simulink model "skidPadSimulation_MPC_Basic"  (R2026a)
settings: Solver=VariableStepAuto  StopTime=80
InitFcn:
  | skidpad_init
values from neighbouring files (symbols this model uses):
  waypoints = [path_data.x_norm, path_data.y_norm, path_data.psi]    [skidpad_init.m]
undefined symbols (not defined in the file or in its folder): ic
settings Model: Creator=lholliday  LastModifiedBy=lholliday

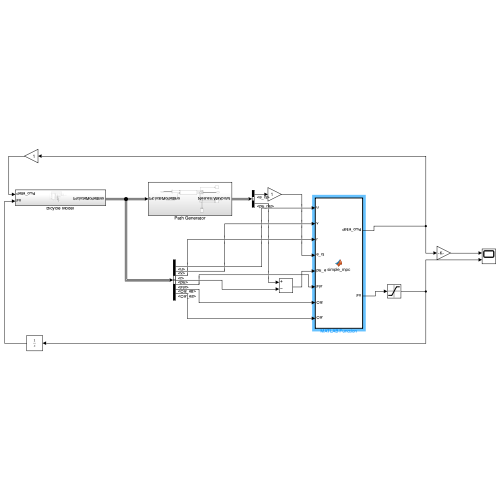
[thumbnail: Simulink's stored preview of the top-level diagram]
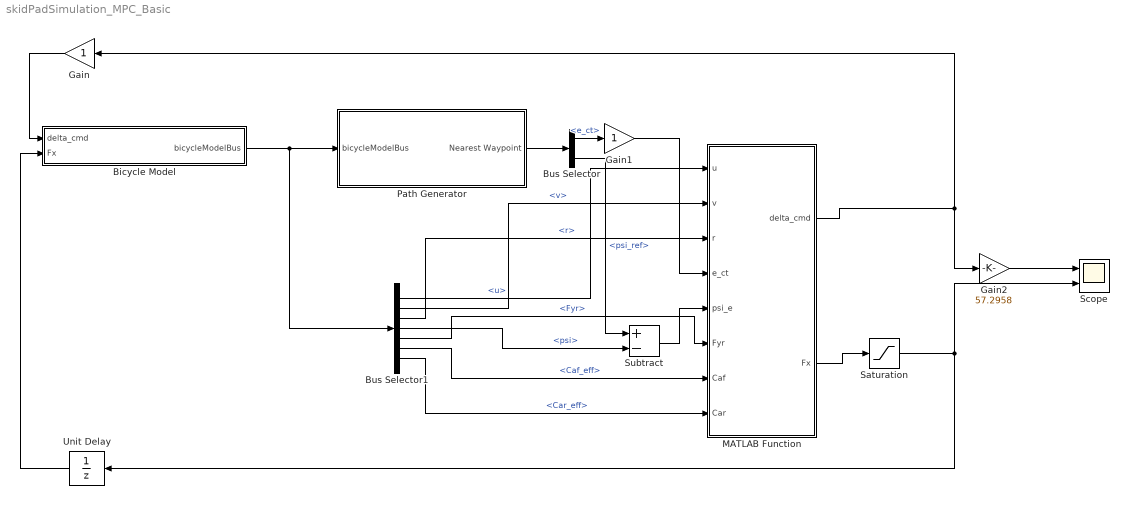
== system skidPadSimulation_MPC_Basic ==
  Bicycle Model : Subsystem
  Bus Selector : BusSelector  OutputSignals=e_ct,psi_ref
  Bus Selector1 : BusSelector  OutputSignals=u,v,r,psi,Fyr,Caf_eff,Car_eff
  Gain : Gain
  Gain1 : Gain
  Gain2 : Gain  Gain=57.2958
  MATLAB Function : MATLAB Function  TreatAsAtomicUnit=on
  Path Generator : Subsystem
  Saturation : Saturate  UpperLimit=2000  LowerLimit=-2000
  Scope : Scope  NumInputPorts=2
      settings: ActiveDisplayYMinimum=-62.500022347760442  ActiveDisplayYMaximum=62.500022347760442  DataLoggingVariableName=ScopeData8
  Subtract : Sum  Inputs=+-
  Unit Delay : UnitDelay  SampleTime=0.01
  wires:
  Path Generator/1(Nearest Waypoint) -> Bus Selector/1
  Bicycle Model/1(bicycleModelBus) -> Path Generator/1(bicycleModelBus), Bus Selector1/1
  Bus Selector/1 -> Gain1/1  "<e_ct>"
  Bus Selector/2 -> Subtract/1  "<psi_ref>"
  Bus Selector1/4 -> Subtract/2  "<psi>"
  Subtract/1 -> MATLAB Function/5(psi_e)
  Bus Selector1/1 -> MATLAB Function/1(u)  "<u>"
  Bus Selector1/2 -> MATLAB Function/2(v)  "<v>"
  Bus Selector1/3 -> MATLAB Function/3(r)  "<r>"
  MATLAB Function/2(Fx) -> Saturation/1
  Bus Selector1/5 -> MATLAB Function/6(Fyr)  "<Fyr>"
  Saturation/1 -> Scope/2, Unit Delay/1
  Gain/1 -> Bicycle Model/1(delta_cmd)
  Gain1/1 -> MATLAB Function/4(e_ct)
  MATLAB Function/1(delta_cmd) -> Gain/1, Gain2/1
  Gain2/1 -> Scope/1
  Unit Delay/1 -> Bicycle Model/2(Fx)
  Bus Selector1/6 -> MATLAB Function/7(Caf)  "<Caf_eff>"
  Bus Selector1/7 -> MATLAB Function/8(Car)  "<Car_eff>"

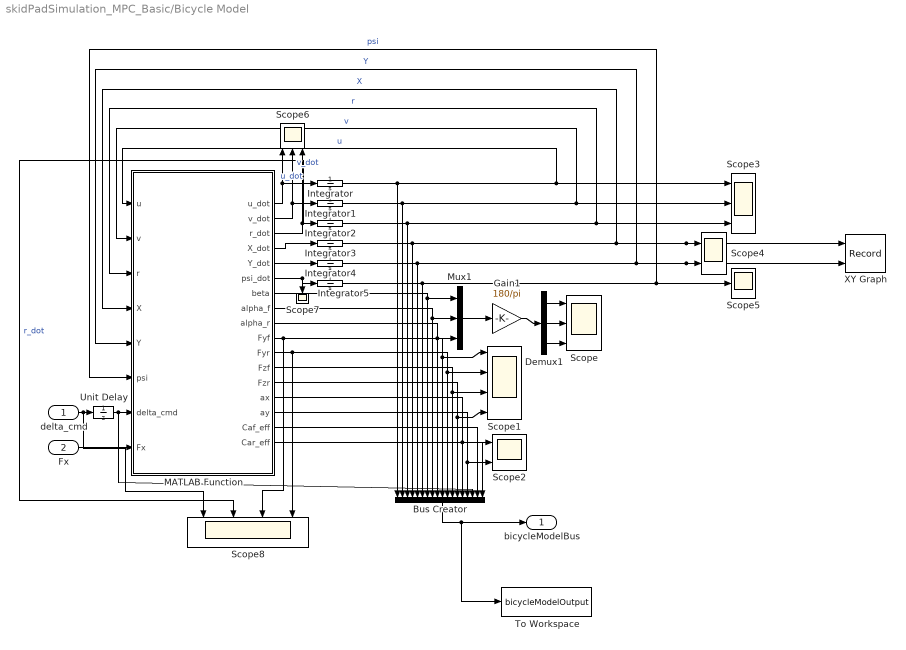
== system skidPadSimulation_MPC_Basic/Bicycle Model ==
  delta_cmd : Inport
  Fx : Inport  Port=2
  Bus Creator : BusCreator  Inputs=18
  Demux1 : Demux  Outputs=3
  Gain1 : Gain  Gain=180/pi
  Integrator : Integrator  InitialCondition=1
  Integrator1 : Integrator
  Integrator2 : Integrator
  Integrator3 : Integrator  InitialCondition=ic.X
  Integrator4 : Integrator  InitialCondition=ic.Y
  Integrator5 : Integrator
  MATLAB Function : MATLAB Function  TreatAsAtomicUnit=on
  Mux1 : Mux  Inputs=3
  Scope : Scope  NumInputPorts=3
      settings: ActiveDisplayYMinimum=-4.6519125249933184  ActiveDisplayYMaximum=6.7259914561440342
  Scope1 : Scope  NumInputPorts=4
      settings: ActiveDisplayYMinimum=-8171.7683750096539  ActiveDisplayYMaximum=8472.1779002535986
  Scope2 : Scope  NumInputPorts=2
      settings: ActiveDisplayYMinimum=-9.4735919080060764  ActiveDisplayYMaximum=10.384655851195211  DataLoggingVariableName=ScopeData2
  Scope3 : Scope  NumInputPorts=3
      settings: ActiveDisplayYMinimum=-0.57485772650992173  ActiveDisplayYMaximum=15.1737195385893  DataLoggingVariableName=ScopeData3
  Scope4 : Scope  NumInputPorts=2
      settings: ActiveDisplayYMinimum=-1031.663648785918  ActiveDisplayYMaximum=2103.4580897021219  DataLoggingVariableName=ScopeData4
  Scope5 : Scope
      settings: ActiveDisplayYMinimum=-1  ActiveDisplayYMaximum=1  DataLoggingVariableName=ScopeData5
  Scope6 : Scope  NumInputPorts=3
      settings: ActiveDisplayYMinimum=-0.28609045005768552  ActiveDisplayYMaximum=2.7161396379868852  DataLoggingVariableName=ScopeData6
  Scope7 : Scope
      settings: ActiveDisplayYMinimum=-1.109696536806452  ActiveDisplayYMaximum=1.2916224827655673  DataLoggingVariableName=ScopeData10
  Scope8 : Scope  NumInputPorts=4
      settings: ActiveDisplayYMinimum=-0.43633231299858238  ActiveDisplayYMaximum=0.43633231299858238  DataLoggingVariableName=ScopeData11
  To Workspace : ToWorkspace  VariableName=bicycleModelOutput  SaveFormat=Timeseries  SampleTime=-1
  Unit Delay : UnitDelay  SampleTime=0.01
  XY Graph : Record  NumPorts=2.0  FileSettingsInternal="{\"entries\":[{\"content\":{\"excelSettings\":{\"content\":{},\"type\":\"Streamout.ExcelSettings\"},\"parquetSettings\":{\"content\":{},\"type\":\"Streamout.ParquetSettings\"}},\"type\":\"Streamout.FileSettingStorage\",\"uuid\":\"\"}],\"packageUris\":[\"http:\\/\\/schema.mathworks.com\\/mf0\\/streamout_blocks\\/R2020a\"],\"version\":\"1.0\"}"  FrameSettings=[0, 0]  Layout=[1 1]  SignalsInternal="{\"entries\":[{\"content\":{\"signals\":[{\"content\":{\"blockPath\":[],\"dimensions\":[1],\"domain\":\"\",\"lineColor\":\"#a2142f\",\"plots\":[ 1 ],\"port\":1,\"sid\":[\"\"],\"signalID\":1,\"signalName\":\"X\"},\"type\":\"RecordBlkView.Signal\",\"uuid\":\"\"},{\"content\":{\"blockPath\":[],\"dimensions\":[1],\"domain\":\"\",\"lineColor\":\"#139fff\",\"plots\":[ 1 ],\"port\":2,\"sid\":[\"\"],\"signalID\":2,\"signalName\":\"Y\"},\"type\":\"RecordBlkView.Signal\",\"uuid\":\"\"}]},\"type\":\"RecordBlkView.InputSignals\",\"uuid\":\"\"}],\"packageUris\":[\"http:\\/\\/schema.mathworks.com\\/mf0\\/streamout_blocks\\/R2020a\"],\"version\":\"1.0\"}"  VisualizationBindings="{\"xyplotplugin\":{\"info\":[{\"series\":[{\"bindingParametersList\":[{\"parameter\":\"X-Axis\",\"signalID\":1,\"signalName\":\"X\"},{\"parameter\":\"Y-Axis\",\"signalID\":2,\"signalName\":\"Y\"}],\"seriesID\":0}],\"subplotID\":1}]}}"  CompatibilityTag=XY
  bicycleModelBus : Outport
  wires:
  ? -> ?
  MATLAB Function/2(v_dot) -> Scope6/2, Integrator1/1  "v_dot"
  MATLAB Function/3(r_dot) -> Scope8/2, Scope6/3, Integrator2/1  "r_dot"
  MATLAB Function/4(X_dot) -> Integrator3/1
  MATLAB Function/5(Y_dot) -> Integrator4/1
  MATLAB Function/6(psi_dot) -> Integrator5/1, Scope7/1
  MATLAB Function/1(u_dot) -> Scope6/1, Integrator/1  "u_dot"
  Integrator1/1 -> Scope3/2, MATLAB Function/2(v), Bus Creator/2  "v"
  Integrator2/1 -> Scope3/3, MATLAB Function/3(r), Bus Creator/3  "r"
  Integrator3/1 -> MATLAB Function/4(X), XY Graph/1, Scope4/1, Bus Creator/4  "X"
  Integrator4/1 -> MATLAB Function/5(Y), XY Graph/2, Scope4/2, Bus Creator/5  "Y"
  Integrator5/1 -> MATLAB Function/6(psi), Scope5/1, Bus Creator/6  "psi"
  MATLAB Function/8(alpha_f) -> Bus Creator/8, Mux1/2
  MATLAB Function/7(beta) -> Bus Creator/7, Mux1/1
  MATLAB Function/10(Fyf) -> Scope8/3, Bus Creator/10, Scope1/1
  MATLAB Function/12(Fzf) -> Bus Creator/12, Scope1/3
  MATLAB Function/13(Fzr) -> Bus Creator/13, Scope1/4
  MATLAB Function/15(ay) -> Scope2/2, Bus Creator/15
  MATLAB Function/14(ax) -> Scope2/1, Bus Creator/14
  Fx/1 -> MATLAB Function/8(Fx)
  Bus Creator/1 -> To Workspace/1, bicycleModelBus/1
  Integrator/1 -> Scope3/1, MATLAB Function/1(u), Bus Creator/1  "u"
  delta_cmd/1 -> Scope8/1, Unit Delay/1
  Unit Delay/1 -> Bus Creator/16, MATLAB Function/7(delta_cmd)
  Gain1/1 -> Demux1/1
  Mux1/1 -> Gain1/1
  Demux1/1 -> Scope/1
  Demux1/2 -> Scope/2
  Demux1/3 -> Scope/3
  MATLAB Function/11(Fyr) -> Scope8/4, Bus Creator/11, Scope1/2
  MATLAB Function/9(alpha_r) -> Bus Creator/9, Mux1/3
  MATLAB Function/16(Caf_eff) -> Bus Creator/17
  MATLAB Function/17(Car_eff) -> Bus Creator/18

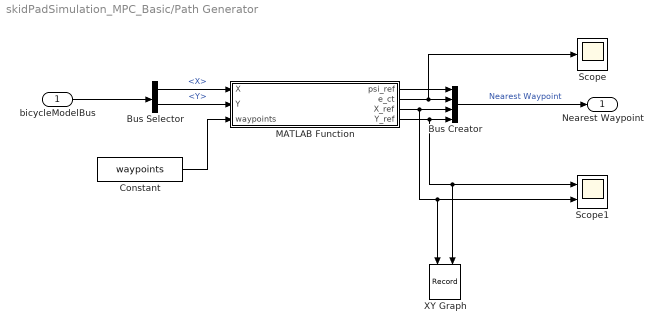
== system skidPadSimulation_MPC_Basic/Path Generator ==
  bicycleModelBus : Inport
  Bus Creator : BusCreator  Inputs=4
  Bus Selector : BusSelector  OutputSignals=X,Y
  Constant : Constant  Value=waypoints
  MATLAB Function : MATLAB Function  TreatAsAtomicUnit=on
  Scope : Scope
      settings: ActiveDisplayYMinimum=-362.12936641992621  ActiveDisplayYMaximum=253.81612411681579  DataLoggingVariableName=ScopeData7
  Scope1 : Scope  NumInputPorts=2
      settings: ActiveDisplayYMinimum=-362.12936641992621  ActiveDisplayYMaximum=253.81612411681579  DataLoggingVariableName=ScopeData9
  XY Graph : Record  NumPorts=2.0  FileSettingsInternal="{\"entries\":[{\"content\":{\"excelSettings\":{\"content\":{},\"type\":\"Streamout.ExcelSettings\"},\"parquetSettings\":{\"content\":{},\"type\":\"Streamout.ParquetSettings\"}},\"type\":\"Streamout.FileSettingStorage\",\"uuid\":\"\"}],\"packageUris\":[\"http:\\/\\/schema.mathworks.com\\/mf0\\/streamout_blocks\\/R2020a\"],\"version\":\"1.0\"}"  FrameSettings=[0, 0]  Layout=[1 1]  SignalsInternal="{\"entries\":[{\"content\":{\"signals\":[{\"content\":{\"blockPath\":[],\"dimensions\":[1],\"domain\":\"\",\"lineColor\":\"#a2142f\",\"plots\":[ 1 ],\"port\":1,\"sid\":[\"\"],\"signalID\":1,\"signalName\":\"MATLAB Function:3\"},\"type\":\"RecordBlkView.Signal\",\"uuid\":\"\"},{\"content\":{\"blockPath\":[],\"dimensions\":[1],\"domain\":\"\",\"lineColor\":\"#139fff\",\"plots\":[ 1 ],\"port\":2,\"sid\":[\"\"],\"signalID\":2,\"signalName\":\"MATLAB Function:4\"},\"type\":\"RecordBlkView.Signal\",\"uuid\":\"\"}]},\"type\":\"RecordBlkView.InputSignals\",\"uuid\":\"\"}],\"packageUris\":[\"http:\\/\\/schema.mathworks.com\\/mf0\\/streamout_blocks\\/R2020a\"],\"version\":\"1.0\"}"  VisualizationBindings="{\"xyplotplugin\":{\"info\":[{\"series\":[{\"bindingParametersList\":[{\"parameter\":\"X-Axis\",\"signalID\":1,\"signalName\":\"MATLAB Function:3\"},{\"parameter\":\"Y-Axis\",\"signalID\":2,\"signalName\":\"MATLAB Function:4\"}],\"seriesID\":0}],\"subplotID\":1}]}}"  CompatibilityTag=XY
  Nearest Waypoint : Outport
  wires:
  bicycleModelBus/1 -> Bus Selector/1
  Bus Selector/1 -> MATLAB Function/1(X)  "<X>"
  Bus Selector/2 -> MATLAB Function/2(Y)  "<Y>"
  MATLAB Function/1(psi_ref) -> Bus Creator/1
  MATLAB Function/2(e_ct) -> Scope/1, Bus Creator/2
  MATLAB Function/3(X_ref) -> XY Graph/1, Scope1/2, Bus Creator/3
  MATLAB Function/4(Y_ref) -> XY Graph/2, Scope1/1, Bus Creator/4
  Bus Creator/1 -> Nearest Waypoint/1  "Nearest Waypoint"
  Constant/1 -> MATLAB Function/3(waypoints)

== matlab function skidPadSimulation_MPC_Basic/Path Generator/MATLAB Function ==
  settings: updateMethod=DISCRETE
  data: X input; psi_ref output; Y input; e_ct output; X_ref output; Y_ref output; waypoints input
function [psi_ref, e_ct, X_ref, Y_ref] = nearest_waypoint(X, Y, waypoints)

% NEAREST_WAYPOINT  Robust path-relative error calculation.
%
% Improvements over basic nearest-point search:
%   1. Persistent forward-only progress index - prevents the index
%      jumping backward or matching a point from a previous lap.
%   2. Bounded local search window around the last known progress -
%      cheaper than scanning all waypoints, and structurally prevents
%      far-away false matches.
%   3. True nearest-point-on-SEGMENT projection (not nearest waypoint) -
%      gives continuous, sub-waypoint-spacing accuracy for e_ct.
%   4. Linear interpolation of psi_ref between the two bracketing
%      waypoints, rather than a discrete jump at each waypoint.
%
% INPUTS:
%   X, Y      - current vehicle position [m]
%   waypoints - [N x 3] array of [X_wp, Y_wp, psi_wp]
%
% OUTPUTS:
%   psi_ref - interpolated path heading at the nearest point [rad]
%   e_ct    - signed cross track error, positive = left of path [m]
%   X_ref   - nearest point ON THE PATH (segment-projected, not a
%             discrete waypoint) [m]
%   Y_ref   - as above [m]

persistent prog_idx
if isempty(prog_idx)
    prog_idx = int32(1);
end

n = int32(size(waypoints, 1));

% -------------------------------------------------------------------
% Step 1: bounded forward search for the nearest waypoint, starting
% from last known progress. Allows a small backward window in case the
% car is briefly behind its last matched point (e.g. low speed,
% momentary correction), but never searches far enough back to match
% a previous lap.
% -------------------------------------------------------------------
back_window = int32(5);
fwd_window  = int32(40);

i_start = max(int32(1), prog_idx - back_window);
i_end   = min(n, prog_idx + fwd_window);

search_idx = i_start:i_end;
dx = waypoints(search_idx,1) - X;
dy = waypoints(search_idx,2) - Y;
dist_sq = dx.^2 + dy.^2;

[~, local_min] = min(dist_sq);
nearest_idx = search_idx(local_min);

prog_idx = nearest_idx;   % advance persistent progress

% -------------------------------------------------------------------
% Step 2: project the vehicle position onto the path SEGMENT either
% side of nearest_idx (whichever segment it actually falls within),
% rather than just using the nearest discrete waypoint. This removes
% most of the e_ct discretisation error from waypoint spacing.
% -------------------------------------------------------------------
idx_prev = max(int32(1), nearest_idx - int32(1));
idx_next = min(n,        nearest_idx + int32(1));

[Xp1, Yp1, dproj1, t1] = project_to_segment(X, Y, waypoints(idx_prev,1:2), waypoints(nearest_idx,1:2));
[Xp2, Yp2, dproj2, t2] = project_to_segment(X, Y, waypoints(nearest_idx,1:2), waypoints(idx_next,1:2));

if dproj1 <= dproj2
    X_ref = Xp1;
    Y_ref = Yp1;
    psi_a = waypoints(idx_prev, 3);
    psi_b = waypoints(nearest_idx, 3);
    t     = t1;
else
    X_ref = Xp2;
    Y_ref = Yp2;
    psi_a = waypoints(nearest_idx, 3);
    psi_b = waypoints(idx_next, 3);
    t     = t2;
end

% -------------------------------------------------------------------
% Step 3: interpolate heading between the two bracketing waypoints
% (shortest-angle interpolation to avoid wraparound issues near +-pi)
% -------------------------------------------------------------------
dpsi = atan2(sin(psi_b - psi_a), cos(psi_b - psi_a));
psi_ref = psi_a + t * dpsi;
psi_ref = atan2(sin(psi_ref), cos(psi_ref));   % wrap to [-pi, pi]

% -------------------------------------------------------------------
% Step 4: signed cross track error using the interpolated path heading
% -------------------------------------------------------------------
dx_ref = X - X_ref;
dy_ref = Y - Y_ref;
e_ct   = -sin(psi_ref)*dx_ref + cos(psi_ref)*dy_ref;

end


function [Xp, Yp, dist_sq, t] = project_to_segment(X, Y, P1, P2)
% Project point (X,Y) onto the segment P1->P2, clamped to [0,1].
% Returns the projected point, squared distance to it, and the
% fractional position t along the segment (used for interpolation).

vx = P2(1) - P1(1);
vy = P2(2) - P1(2);
seg_len_sq = vx^2 + vy^2;

if seg_len_sq < 1e-9
    % Degenerate segment (coincident points) - just use P1
    Xp = P1(1);
    Yp = P1(2);
    t  = 0;
else
    t = ((X - P1(1))*vx + (Y - P1(2))*vy) / seg_len_sq;
    t = max(0, min(1, t));
    Xp = P1(1) + t*vx;
    Yp = P1(2) + t*vy;
end

dist_sq = (X - Xp)^2 + (Y - Yp)^2;

end

== matlab function skidPadSimulation_MPC_Basic/Bicycle Model/MATLAB Function ==
  data: u_dot output; v_dot output; u input; v input; r_dot output; X_dot output; r input; X input; Y input; psi input; delta_cmd input; Fx input; Y_dot output; psi_dot output; beta output; alpha_f output; alpha_r output; Fyf output; Fyr output; Fzf output; Fzr output; ax output; ay output; Caf_eff output; Car_eff output
function [u_dot, v_dot, r_dot, X_dot, Y_dot, psi_dot, ...
          beta, alpha_f, alpha_r, Fyf, Fyr, Fzf, Fzr, ax, ay, Caf_eff, Car_eff] = ...
    bicycle_model_plant(u, v, r, X, Y, psi, delta_cmd, Fx)

% BICYCLE_MODEL_PLANT Nonlinear 6-DOF bicycle model with Pacejka tyres.
%
% FIX (this version): the slip angle clamp previously OVERWROTE alpha_f/
% alpha_r before they were used anywhere else, meaning the equations of
% motion saw a false, capped slip angle even when the tyre was actually
% sliding further. That made the plant internally inconsistent once slip
% exceeded the clamp.
%
% This version keeps the TRUE alpha_f/alpha_r for everything (outputs,
% equations of motion via Fyf/Fyr), and only clamps the SLIP ANGLE INPUT
% TO PACEJKA, i.e. it limits how far out on the curve we evaluate force,
% without lying about what the slip angle actually was. This also adds
% Caf_eff/Car_eff outputs - the local slope of the Pacejka curve at the
% (clamped) operating point - so an external controller (e.g. simple_mpc)
% can use a gain-scheduled effective cornering stiffness instead of a
% fixed constant.
%
% INPUTS:
%   u         - Longitudinal velocity [m/s]
%   v         - Lateral velocity [m/s]
%   r         - Yaw rate [rad/s]
%   X, Y      - Global position [m]
%   psi       - Heading [rad]
%   delta_cmd - Front wheel steer angle [rad]
%   Fx        - Longitudinal force at rear axle [N]
%
% OUTPUTS:
%   u_dot, v_dot, r_dot     - Derivatives of velocities [m/s^2, rad/s^2]
%   X_dot, Y_dot, psi_dot   - Derivatives of position and heading
%   beta                     - Body slip angle [rad]
%   alpha_f, alpha_r         - TRUE front and rear slip angles [rad]
%                              (NOT clamped - this is the real value)
%   Fyf, Fyr                 - Front and rear lateral tyre forces [N]
%                              (computed from a slip angle clamped only
%                              for the Pacejka EVALUATION, see below)
%   Fzf, Fzr                 - Front and rear normal loads [N]
%   ax, ay                   - Longitudinal and lateral accelerations [m/s^2]
%   Caf_eff, Car_eff          - Effective (local-slope) cornering
%                              stiffness at the current operating point
%                              [N/rad]. For use by a gain-scheduled
%                              linear controller.

veh.m    = 1300;
veh.L    = 2.750;
veh.a    = 1.468;
veh.b    = 2.750 - 1.468;
veh.Iz   = 1850;
veh.h_cg = 0.45;
veh.mu   = 1.0;
veh.g    = 9.81;

m    = veh.m;
L    = veh.L;
a    = veh.a;
b    = veh.b;
Iz   = veh.Iz;
mu   = veh.mu;
g    = veh.g;

tyre.f.B = 10.0;
tyre.f.C = 1.9;
tyre.f.E = 0.97;

tyre.r.B = 10.0;
tyre.r.C = 1.9;
tyre.r.E = 0.97;

% -------------------------------------------------------------------------
% Normal Loads (static, no roll dynamics)
% -------------------------------------------------------------------------
Fzf = m * g * b / L;
Fzr = m * g * a / L;

% -------------------------------------------------------------------------
% TRUE Slip Angles - never overwritten, used for all outputs/diagnostics
% -------------------------------------------------------------------------
u_safe = max(u, 0.1);

alpha_f = delta_cmd - atan2(v + a*r, u_safe);
alpha_r = -atan2(v - b*r, u_safe);

% -------------------------------------------------------------------------
% Slip angle CLAMPED ONLY FOR PACEJKA EVALUATION - this limits how far
% out on the tyre curve we evaluate (reasonable, since Pacejka's own
% curvature factor E already handles realistic saturation/falloff, but
% an explicit cap adds a safety margin against numerical extremes at
% very large slip). The TRUE alpha_f/alpha_r above are what's reported
% and what physically happened - this clamp only affects what force
% value we use going forward, exactly like real tyre saturation does.
% -------------------------------------------------------------------------
alpha_max = deg2rad(12);   % wider than 5deg - this is now a safety
                            % bound, not a normal-operation limit
alpha_f_eval = sign(alpha_f) * min(abs(alpha_f), alpha_max);
alpha_r_eval = sign(alpha_r) * min(abs(alpha_r), alpha_max);

% -------------------------------------------------------------------------
% Pacejka Magic Formula Lateral Tyre Forces
% -------------------------------------------------------------------------
Fyf = pacejka_force(rad2deg(alpha_f_eval), Fzf, tyre.f.B, tyre.f.C, tyre.f.E, mu);
Fyr = pacejka_force(rad2deg(alpha_r_eval), Fzr, tyre.r.B, tyre.r.C, tyre.r.E, mu);

% -------------------------------------------------------------------------
% Effective cornering stiffness - local slope of Pacejka curve at the
% current operating point, via small finite difference. Used externally
% by a gain-scheduled linear controller instead of a fixed Caf/Car.
% -------------------------------------------------------------------------
dA = deg2rad(0.5);   % small perturbation for finite difference [rad]

Fyf_p = pacejka_force(rad2deg(alpha_f_eval + dA), Fzf, tyre.f.B, tyre.f.C, tyre.f.E, mu);
Fyf_m = pacejka_force(rad2deg(alpha_f_eval - dA), Fzf, tyre.f.B, tyre.f.C, tyre.f.E, mu);
Caf_eff = abs((Fyf_p - Fyf_m) / (2*dA));

Fyr_p = pacejka_force(rad2deg(alpha_r_eval + dA), Fzr, tyre.r.B, tyre.r.C, tyre.r.E, mu);
Fyr_m = pacejka_force(rad2deg(alpha_r_eval - dA), Fzr, tyre.r.B, tyre.r.C, tyre.r.E, mu);
Car_eff = abs((Fyr_p - Fyr_m) / (2*dA));

% Floor to avoid feeding a near-zero stiffness into a controller (which
% would make the linear model think steering has almost no effect)
Caf_eff = max(Caf_eff, 1000);
Car_eff = max(Car_eff, 1000);

% -------------------------------------------------------------------------
% Equations of Motion (Body Frame) - uses Fyf/Fyr from the (safety-)
% clamped evaluation, which is correct: this IS the real force the tyre
% produces, since real tyres also saturate/fall off at high slip.
% -------------------------------------------------------------------------
u_dot = (Fx - Fyf*sin(delta_cmd))/m + v*r;
v_dot = (Fyf*cos(delta_cmd) + Fyr)/m - u*r;
r_dot = (a*Fyf*cos(delta_cmd) - b*Fyr) / Iz;

% -------------------------------------------------------------------------
% Kinematics (Global Frame)
% -------------------------------------------------------------------------
X_dot   = u*cos(psi) - v*sin(psi);
Y_dot   = u*sin(psi) + v*cos(psi);
psi_dot = r;

% -------------------------------------------------------------------------
% Body Slip Angle
% -------------------------------------------------------------------------
beta = atan2(v, u_safe);

% -------------------------------------------------------------------------
% Accelerations
% -------------------------------------------------------------------------
ax = u_dot;
ay = v_dot + u*r;

end

% =========================================================================
% PACEJKA_FORCE
% =========================================================================
function Fy = pacejka_force(alpha, Fz, B, C, E, mu)
D = mu * Fz;
Balpha        = B * alpha;
arctan_Balpha = atan(Balpha);
inner_arg     = Balpha - E * (Balpha - arctan_Balpha);
Fy            = D * sin(C * atan(inner_arg));
end

== matlab function skidPadSimulation_MPC_Basic/MATLAB Function ==
  data: u input; delta_cmd output; v input; r input; e_ct input; psi_e input; Fyr input; Fx output; Caf input; Car input
function [delta_cmd, Fx] = simple_mpc(u, v, r, e_ct, psi_e, Fyr, Caf, Car)

% SIMPLE_MPC  Minimal linear MPC, closed-form solve, no toolboxes.
%
% State: x = [e_ct; v; psi_e; r]   (raw plant states, NOT their derivatives)
% Control: w = [delta]
%
% This version correctly derives A,B for THIS state definition directly
% from the bicycle model equations of motion, rather than reusing a
% different (rate-based) error-state formulation. State order matches
% exactly what is physically measured: e_ct, v, psi_e, r.
%
% INPUTS:
%   u      - longitudinal speed [m/s]
%   v      - lateral velocity [m/s]
%   r      - yaw rate [rad/s]
%   e_ct   - cross track error [m]
%   psi_e  - heading error = psi_ref - psi [rad]
%   Fyr    - rear lateral tyre force [N]  (used for speed/Fx, not steering)
%
% OUTPUTS:
%   delta_cmd - steer angle [rad]
%   Fx        - longitudinal force [N]

% -------------------------------------------------------------------------
% Fixed vehicle parameters
% -------------------------------------------------------------------------
m   = 1300;
Iz  = 1850;
a   = 1.468;
b   = 1.282;
Caf = 171887;
Car = 171887;
L   = a + b;

u_safe = max(u, 1.0);

% -------------------------------------------------------------------------
% Derive A, B directly for state x = [e_ct; v; psi_e; r]
%
% Bicycle model (small angle, body-frame lateral dynamics):
%   v_dot   = -(2Caf+2Car)/(m*u)*v + (-u + (-2Caf*a+2Car*b)/(m*u))*r + (2Caf/m)*delta
%   r_dot   = (-2Caf*a+2Car*b)/(Iz*u)*v + (-2Caf*a^2-2Car*b^2)/(Iz*u)*r + (2Caf*a/Iz)*delta
%
% Path error kinematics (small angle):
%   e_ct_dot  = v + u*psi_e          (lateral velocity in path frame)
%   psi_e_dot = r - kappa*u          (kappa = path curvature; treated as
%                                      an exogenous disturbance, not a
%                                      state - omitted from A, acceptable
%                                      since horizon is short and curvature
%                                      is slowly varying relative to dt)
% -------------------------------------------------------------------------

A21 = -(2*Caf + 2*Car) / (m*u_safe);
A23 = 0;
A24 = -u_safe + (-2*Caf*a + 2*Car*b) / (m*u_safe);

A41 = 0;
A42 = (-2*Caf*a + 2*Car*b) / (Iz*u_safe);
A44 = (-2*Caf*a^2 - 2*Car*b^2) / (Iz*u_safe);

A = [0,    1,    u_safe,  0;
     0,  A21,    0,     A24;
     0,    0,    0,      1;
     0,  A42,    0,    A44];

B = [0;
     2*Caf/m;
     0;
     2*Caf*a/Iz];

% -------------------------------------------------------------------------
% Discretise (forward Euler)
% -------------------------------------------------------------------------
dt = 0.05;
N  = 5;

Ad = eye(4) + A*dt;
Bd = B*dt;

% -------------------------------------------------------------------------
% Batch prediction matrices
% -------------------------------------------------------------------------
nx = 4;
nu = 1;

Sx = zeros(nx*N, nx);
Su = zeros(nx*N, nu*N);

Ad_pow = eye(nx);
for k = 1:N
    Ad_pow = Ad_pow * Ad;
    Sx((k-1)*nx+1:k*nx, :) = Ad_pow;
end

for k = 1:N
    for jcol = 1:k
        Ad_p = eye(nx);
        for p = 1:(k-jcol)
            Ad_p = Ad_p * Ad;
        end
        Su((k-1)*nx+1:k*nx, jcol) = Ad_p * Bd;
    end
end

% -------------------------------------------------------------------------
% Cost weights - state order [e_ct, v, psi_e, r]
% -------------------------------------------------------------------------
Qdiag = [20000, 1, 200, 1];
Rval  = 5;

Q = kron(eye(N), diag(Qdiag));
R = kron(eye(N), Rval);

% -------------------------------------------------------------------------
% Closed-form unconstrained solve
% -------------------------------------------------------------------------
x0 = [e_ct; v; psi_e; r];

H = Su'*Q*Su + R;
f = Su'*Q*Sx*x0;

W = -H \ f;

delta_raw = W(1);

% -------------------------------------------------------------------------
% Clip steer
% -------------------------------------------------------------------------
delta_max = 50*pi/180;
delta_cmd = max(min(delta_raw, delta_max), -delta_max);

% -------------------------------------------------------------------------
% Speed - always demand max available longitudinal force given current
% lateral tyre force (friction-circle, instantaneous, no horizon needed)
% -------------------------------------------------------------------------
mu  = 1.0;
g   = 9.81;
Fzr = m*g*a/L;

Fx_max_now = sqrt(max(0, (mu*Fzr)^2 - Fyr^2));
Fx = Fx_max_now;

end
